simulink model "PMSM_PI_CONTROL"  (R2024b)
settings: Solver=ode4  StartTime=0.0  StopTime=2  FixedStep=Ts  RelTol=1e-3
InitFcn:
  | p=4;
  | RS=0.9585;
  | Rs=0.9585;
  | LS=0.00525;
  | Lq= 0.00525;
  | LAMDA_F=0.1827;
  | Ld=0.00525;
  | B=0.0003035;
  | J=0.0006329;
  | Vdc=300;
  | vcarp=150;
  | G=Vdc/(2*vcarp);
  | Ts = 1e-6;
  | kpi=2;
  | kii=100;
  | %% Current-loop bandwidth
  | f_ci = 100;        % Current controller bandwidth [Hz]
  | w_ci = 2*pi*f_ci;
  | 
  | %% d-axis PI
  | Kpd = Ld*w_ci;
  | Kid = Rs*w_ci;
  | 
  | %% q-axis PI
  | Kpq = Lq*w_ci;
  | Kiq = Rs*w_ci;
values from neighbouring files (symbols this model uses):
  phase = squeeze(phase)    [fir_filter.m]
  V = VPH - mean(VPH)    [three_level_inverter.m]
libraries: spsdq0toabcLib x2, spsabctoAlphaBetaZeroLib x2, spsabctodq0Lib x1, spsPermanentMagnetSynchronousMachineLib x1, spspowerguiLib x1, slpidlib x1
settings Model: SimulationMode=accelerator  Creator=killa  LastModifiedBy=killa

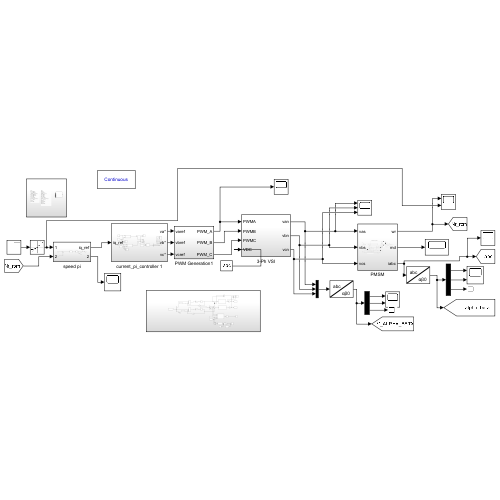
[thumbnail: Simulink's stored preview of the top-level diagram]
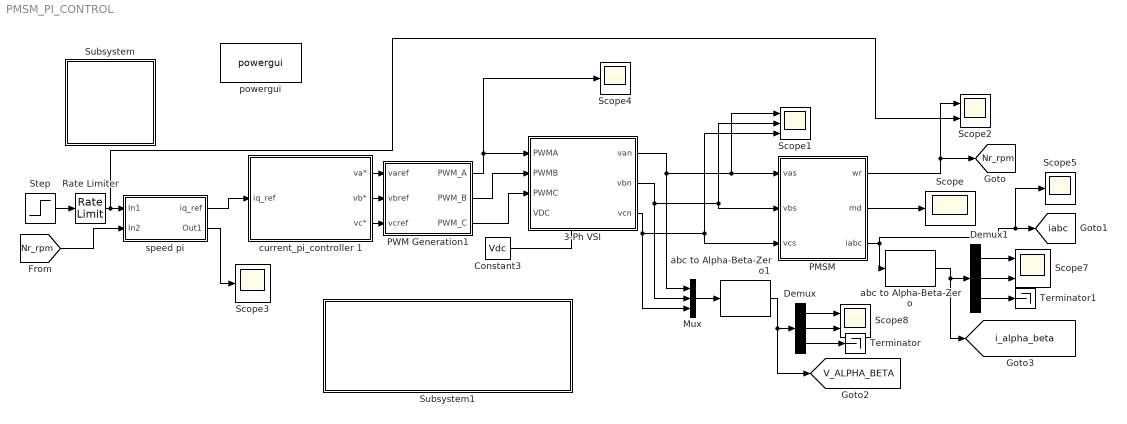
== system PMSM_PI_CONTROL ==
  3-Ph VSI : Subsystem
  Constant3 : Constant  Value=Vdc
  Demux : Demux  Outputs=3
  Demux1 : Demux  Outputs=3
  Mux : Mux  Inputs=3
  PMSM : Subsystem
  PWM Generation1 : Subsystem
  Rate Limiter : RateLimiter  RisingSlewLimit=10000  FallingSlewLimit=-10000
  Scope{,3..5} (4 alike) : Scope
  Scope1 : Scope  NumInputPorts=3
  Scope2 : Scope  NumInputPorts=2
  Scope7 : Scope  NumInputPorts=2
  Scope8 : Scope  NumInputPorts=2
  Step : Step  Before=500  After=1000  SampleTime=0
  Subsystem : Subsystem
  Subsystem1 : Subsystem
  Terminator : Terminator
  Terminator1 : Terminator
  abc to Alpha-Beta-Zero : spsabctoAlphaBetaZeroLib/abc to Alpha-Beta-Zero
  abc to Alpha-Beta-Zero1 : spsabctoAlphaBetaZeroLib/abc to Alpha-Beta-Zero
  current_pi_controller 1 : Subsystem
  powergui : spspowerguiLib/powergui  Priority=1  SimulationMode=Continuous  SampleTime=50e-6  frequency=60  Iterations=50  frequencyindice=60  Pbase=100e6  ErrMax=1e-4  UnitsV=kV  UnitsW=MW  buscounter=0  FunctionMessages=off  echomessages=off  EnableUseOfTLC=off  CurrentSourceSwitches=off  DisableSnubberDevices=off  DisableRonSwitches=off  DisableVfSwitches=off  DisplayEquations=off  AutomaticDiscreteSolvers=off  SolverType=Tustin/Backward Euler (TBE)  Interpol=off  ExternalGateDelay=off  methode=off  Ts=100  x0status=blocks  SPID=on  SwTol=0  HookPort=off  NonlinearTolerance=1e-4  nMaxIteration=100  ContinueOnMaxIteration=off  RestoreLinks=warning  ResistiveCurrentMeasurement=off  Frange=[0:2:500]  Ylog=off  Xlog=on  ShowGrid=off  save=off  variable=ZData  structure=0  ZoomFFT=off  StartTime=0.0  cycles=1  DisplayStyle=1  fundamental=60  FreqAxis=off  MaxFrequency=1000  frequencyindicesteady=1  RmsSteady=1  display=off
  speed pi : Subsystem
  tag scope: Nr_rpm=global, V_ALPHA_BETA=global, i_alpha_beta=global, iabc=global
  wires:
  PWM Generation1/1(PWM_A) -> Scope4/1, 3-Ph VSI/1(PWMA)
  speed pi/1(iq_ref) -> current_pi_controller 1/1(iq_ref)
  speed pi/2(Out1) -> Scope3/1
  Step/1 -> Rate Limiter/1
  Constant3/1 -> 3-Ph VSI/4(VDC)
  [Nr_rpm] -> speed pi/2(In2)
  PMSM/1(wr) -> [Nr_rpm], Scope2/1
  3-Ph VSI/3(vcn) -> Mux/3, PMSM/3(vcs), Scope1/3
  PWM Generation1/3(PWM_C) -> 3-Ph VSI/3(PWMC)
  PWM Generation1/2(PWM_B) -> 3-Ph VSI/2(PWMB)
  3-Ph VSI/1(van) -> PMSM/1(vas), Scope1/1, Mux/1
  current_pi_controller 1/1(va*) -> PWM Generation1/1(varef)
  current_pi_controller 1/3(vc*) -> PWM Generation1/3(vcref)
  current_pi_controller 1/2(vb*) -> PWM Generation1/2(vbref)
  PMSM/3(iabc) -> Scope5/1, [iabc], abc to Alpha-Beta-Zero/1
  PMSM/2(md) -> Scope/1
  Mux/1 -> abc to Alpha-Beta-Zero1/1
  3-Ph VSI/2(vbn) -> Mux/2, PMSM/2(vbs), Scope1/2
  Demux/1 -> Scope8/1
  Demux/2 -> Scope8/2
  abc to Alpha-Beta-Zero/1 -> [i_alpha_beta], Demux1/1
  Demux1/1 -> Scope7/1
  Demux1/2 -> Scope7/2
  Demux/3 -> Terminator/1
  Demux1/3 -> Terminator1/1
  abc to Alpha-Beta-Zero1/1 -> [V_ALPHA_BETA], Demux/1
  Rate Limiter/1 -> Scope2/2, speed pi/1(In1)

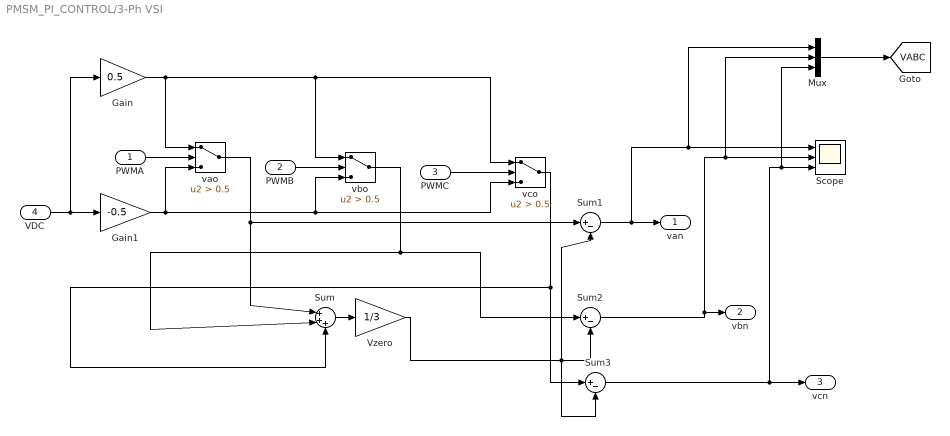
== system PMSM_PI_CONTROL/3-Ph VSI ==
  PWMA : Inport
  PWMB : Inport  Port=2
  PWMC : Inport  Port=3
  VDC : Inport  Port=4
  Gain : Gain  Gain=0.5
  Gain1 : Gain  Gain=-0.5
  Mux : Mux  Inputs=3
  Scope : Scope  NumInputPorts=3
  Sum : Sum  Inputs=|+++
  Sum1 : Sum  Inputs=|+-
  Sum2 : Sum  Inputs=|+-
  Sum3 : Sum  Inputs=|+-
  Vzero : Gain  Gain=1/3
  vao : Switch  Criteria=u2 > Threshold  Threshold=0.5  SaturateOnIntegerOverflow=off  InputSameDT=off
  vbo : Switch  Criteria=u2 > Threshold  Threshold=0.5  SaturateOnIntegerOverflow=off  InputSameDT=off
  vco : Switch  Criteria=u2 > Threshold  Threshold=0.5  SaturateOnIntegerOverflow=off  InputSameDT=off
  van : Outport
  vbn : Outport  Port=2
  vcn : Outport  Port=3
  tag scope: VABC=global
  wires:
  Gain/1 -> vao/1, vbo/1, vco/1
  Gain1/1 -> vao/3, vbo/3, vco/3
  VDC/1 -> Gain/1, Gain1/1
  PWMA/1 -> vao/2
  PWMB/1 -> vbo/2
  PWMC/1 -> vco/2
  vbo/1 -> Sum/2, Sum2/1
  vco/1 -> Sum/3, Sum3/1
  Sum/1 -> Vzero/1
  vao/1 -> Sum/1, Sum1/1
  Sum1/1 -> Mux/1, Scope/1, van/1
  Sum2/1 -> Mux/2, Scope/2, vbn/1
  Sum3/1 -> Mux/3, Scope/3, vcn/1
  Vzero/1 -> Sum3/2, Sum2/2, Sum1/2
  Mux/1 -> [VABC]

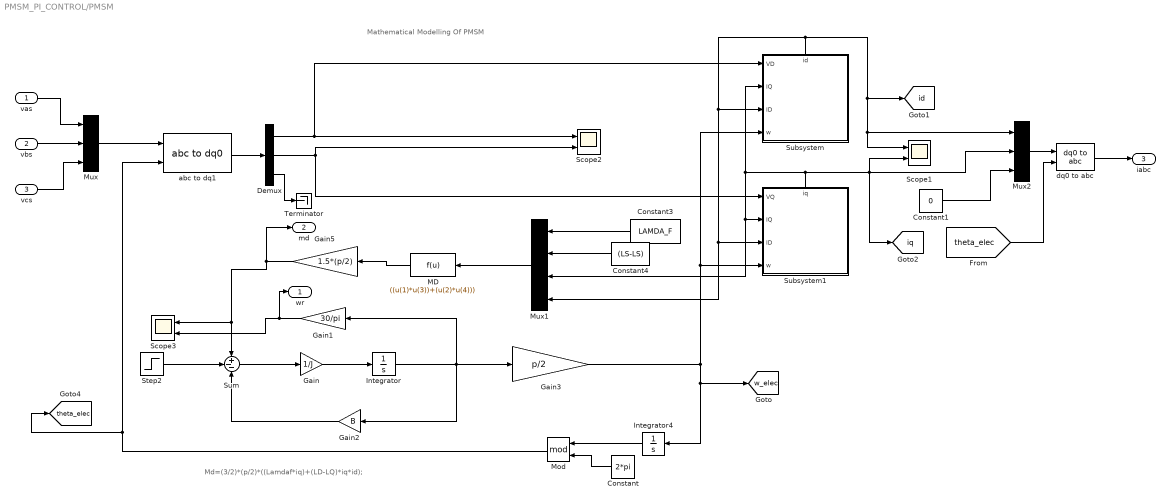
== system PMSM_PI_CONTROL/PMSM ==
  note: Mathematical Modelling Of PMSM
  note: Md=(3/2)*(p/2)*((Lamdaf*iq)+(LD-LQ)*iq*id);
  vas : Inport
  vbs : Inport  Port=2
  vcs : Inport  Port=3
  Constant : Constant  Value=2*pi
  Constant1 : Constant  Value=0
  Constant3 : Constant  Value=LAMDA_F
  Constant4 : Constant  Value=(LS-LS)
  Demux : Demux  Outputs=3
  Gain : Gain  Gain=1/J
  Gain1 : Gain  Gain=30/pi
  Gain2 : Gain  Gain=B
  Gain3 : Gain  Gain=p/2
  Gain5 : Gain  Gain=1.5*(p/2)
  Integrator : Integrator
  Integrator4 : Integrator
  MD : Fcn  Expr=((u(1)*u(3))+(u(2)*u(4)))
  Mod : Math  Operator=mod
  Mux : Mux  Inputs=3
  Mux1 : Mux
  Mux2 : Mux  Inputs=3
  Scope1 : Scope  NumInputPorts=2
  Scope2 : Scope  NumInputPorts=2
  Scope3 : Scope  NumInputPorts=2
  Step2 : Step  Time=0.5  Before=1  After=5  SampleTime=0
  Subsystem : Subsystem
      settings: PortSchema="{\"entries\":[{\"content\":{\"sides\":[{\"content\":{\"connectorIds\":[\"In1\",\"In2\",\"In3\",\"In4\"]},\"type\":\"ConnectorPlacement.EquallySpacedRectSide\",\"uuid\":\"8bdfacbe-4a3a-4ee8-bd8b-fd9f165566ad\"},{\"content\":{\"side\":\"RIGHT\"},\"type\":\"ConnectorPlacement.EquallySpacedRectSide\",\"uuid\":\"d7d447ea-68c0-4048-9ad9-b0a4b9da88db\"},{\"content\":{\"connectorIds\":[\"Out1\"],\"side\":\"TOP\"},\"type\":\"ConnectorPlacement.EquallySpacedRectSide\",\"uuid\":\"b7ac2ad5-65e5-4d40-8b7d-b38f0c69dbd3\"}]},\"type\":\"ConnectorPlacement.EquallySpacedConnector\",\"uuid\":\"b233c12a-b13d-4732-89f8-f9fe229221af\"}],\"packageUris\":[\"http://schema.mathworks.com/mf0/Connector/R2020b\"],\"version\":\"1.0\"}"
  Subsystem1 : Subsystem
      settings: PortSchema="{\"entries\":[{\"content\":{\"sides\":[{\"content\":{\"connectorIds\":[\"In1\",\"In2\",\"In3\",\"In4\"]},\"type\":\"ConnectorPlacement.EquallySpacedRectSide\",\"uuid\":\"6a02ce95-2547-4019-ba1c-0297980e75c1\"},{\"content\":{\"side\":\"RIGHT\"},\"type\":\"ConnectorPlacement.EquallySpacedRectSide\",\"uuid\":\"b1a391f9-ac05-4a60-810a-c34cda090cbe\"},{\"content\":{\"connectorIds\":[\"Out1\"],\"side\":\"TOP\"},\"type\":\"ConnectorPlacement.EquallySpacedRectSide\",\"uuid\":\"b02dfd25-1f32-4ddc-a79d-3ed5d594643e\"}]},\"type\":\"ConnectorPlacement.EquallySpacedConnector\",\"uuid\":\"98d8064c-9ae1-4c8d-8330-54a5e7664553\"}],\"packageUris\":[\"http://schema.mathworks.com/mf0/Connector/R2020b\"],\"version\":\"1.0\"}"
  Sum : Sum  Inputs=+--
  Terminator : Terminator
  abc to dq1 : spsabctodq0Lib/abc to dq0  Alignment=90 degrees behind phase A axis
  dq0 to abc : spsdq0toabcLib/dq0 to abc  Alignment=90 degrees behind phase A axis
  wr : Outport
  md : Outport  Port=2
  iabc : Outport  Port=3
  tag scope: id=global, iq=global, theta_elec=global, w_elec=global
  wires:
  Gain3/1 -> [w_elec], Integrator4/1, Subsystem/4(w), Subsystem1/4(w)
  Gain1/1 -> wr/1, Scope3/2
  Subsystem/1(id) -> [id], Mux2/1, Scope1/1, Mux1/4, Subsystem1/3(ID), Subsystem/3(ID)
  Gain2/1 -> Sum/3
  Demux/1 -> Scope2/1, Subsystem/1(VD)
  abc to dq1/1 -> Demux/1
  Step2/1 -> Sum/2
  Integrator/1 -> Gain2/1, Gain3/1, Gain1/1
  Subsystem1/1(iq) -> [iq], Mux2/2, Scope1/2, Subsystem/2(IQ), Mux1/3, Subsystem1/2(IQ)
  Integrator4/1 -> Mod/1
  Constant3/1 -> Mux1/1
  MD/1 -> Gain5/1
  Mux1/1 -> MD/1
  Constant/1 -> Mod/2
  Demux/3 -> Terminator/1
  Gain5/1 -> Scope3/1, Sum/1, md/1
  Gain/1 -> Integrator/1
  Sum/1 -> Gain/1
  Demux/2 -> Scope2/2, Subsystem1/1(VQ)
  Constant4/1 -> Mux1/2
  Mux/1 -> abc to dq1/1
  vas/1 -> Mux/1
  vbs/1 -> Mux/2
  vcs/1 -> Mux/3
  Mux2/1 -> dq0 to abc/1
  Constant1/1 -> Mux2/3
  [theta_elec] -> dq0 to abc/2
  dq0 to abc/1 -> iabc/1
  Mod/1 -> [theta_elec], abc to dq1/2

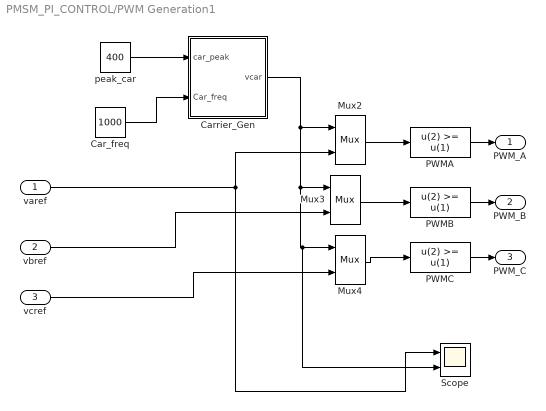
== system PMSM_PI_CONTROL/PWM Generation1 ==
  varef : Inport
  vbref : Inport  Port=2
  vcref : Inport  Port=3
  Car_freq : Constant  Value=1000
  Carrier_Gen : Subsystem
  Mux2 : Mux  Inputs=2
  Mux3 : Mux  Inputs=2
  Mux4 : Mux  Inputs=2
  PWMA : Fcn  Expr=u(2) >= u(1)
  PWMB : Fcn  Expr=u(2) >= u(1)
  PWMC : Fcn  Expr=u(2) >= u(1)
  Scope : Scope  NumInputPorts=2
  peak_car : Constant  Value=400
  PWM_A : Outport
  PWM_B : Outport  Port=2
  PWM_C : Outport  Port=3
  wires:
  varef/1 -> Mux2/2, Scope/1
  Car_freq/1 -> Carrier_Gen/2(Car_freq)
  peak_car/1 -> Carrier_Gen/1(car_peak)
  vcref/1 -> Mux4/2
  PWMC/1 -> PWM_C/1
  vbref/1 -> Mux3/2
  PWMB/1 -> PWM_B/1
  PWMA/1 -> PWM_A/1
  Mux4/1 -> PWMC/1
  Mux3/1 -> PWMB/1
  Mux2/1 -> PWMA/1
  Carrier_Gen/1(vcar) -> Mux2/1, Mux3/1, Mux4/1, Scope/2

== system PMSM_PI_CONTROL/Subsystem ==
  note: p=4;
      | RS=0.9585;
      | LS=0.00525;
      | LAMDA_F=0.1827;
      | B=0.0003035;
      | J=0.0006329;
      | Vdc=300;
      | vcarp=150;
      | G=Vdc/(2*vcarp);
      | Ts = 1e-6;
      | kpi=2;
      | kii=100;
  note: p=8;
      | RS=30;
      | LS=50e-3;
      | LAMDA_F=0.2;
      | B=0.0003;
      | J=0.002;
      | Vdc=400;
      | vcarp=150;
      | G=Vdc/(2*vcarp);
      | Ts = 1e-6;
      | kpid=2;
      | kiid=100;
      | kpiq=2;
      | kiiq=100;
  Permanent Magnet Synchronous Machine : spsPermanentMagnetSynchronousMachineLib/Permanent Magnet Synchronous Machine  Commented=on  NbPhases=3  FluxDistribution=Sinusoidal  RotorType=Round  MechanicalLoad=Torque Tm  PresetModel="05:  8 Nm 300 Vdc 2000 RPM - 10 Nm"  ShowDetailedParameters=on  MeasurementBus=off  Resistance=0.9585  Inductance=8.5e-3  dqInductances=[8.5e-3,8.5e-3]  La=0.00525  MachineConstant=Flux linkage established by magnets (V.s)  Flux=0.1827  VoltageCst=132.5525  TorqueCst=1.0962  Flat=120  Mechanical=[0.0006329 0.0003035 4 0]  PolePairs=4  InitialConditions=[0,0, 0,0]  InitialConditions5ph=[0 0 0 0 0 0]  RefAngle=90 degrees behind phase A axis (modified Park)  IterativeDiscreteModel=Trapezoidal non iterative  TsBlock=-1  TsPowergui=0

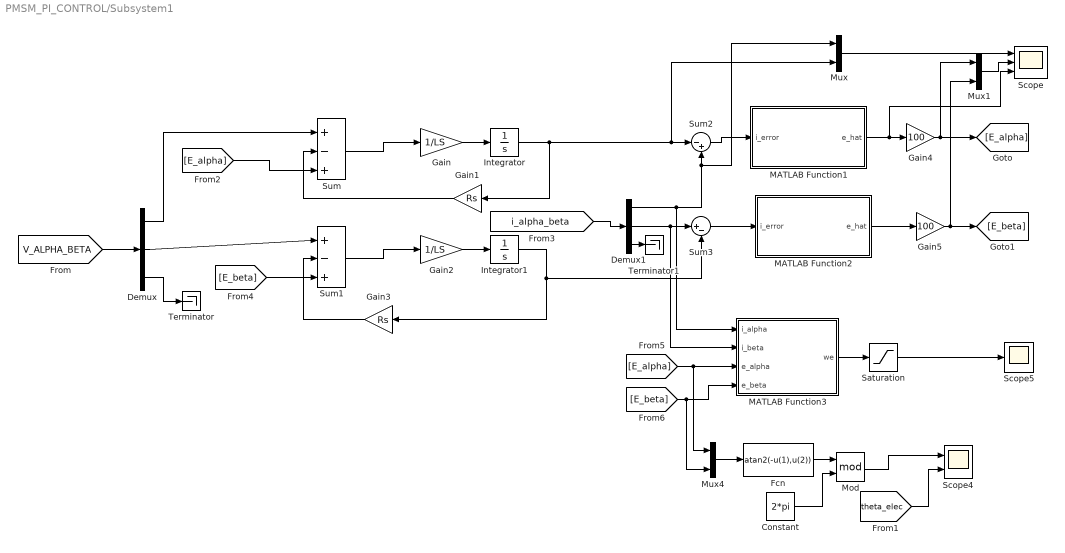
== system PMSM_PI_CONTROL/Subsystem1 ==
  Constant : Constant  Value=2*pi
  Demux : Demux  Outputs=3
  Demux1 : Demux  Outputs=3
  Fcn : Fcn  Expr=atan2(-u(1),u(2))
  Gain : Gain  Gain=1/LS
  Gain1 : Gain  Gain=Rs
  Gain2 : Gain  Gain=1/LS
  Gain3 : Gain  Gain=Rs
  Gain4 : Gain  Gain=100
  Gain5 : Gain  Gain=100
  Integrator : Integrator
  Integrator1 : Integrator
  MATLAB Function1 : MATLAB Function  TreatAsAtomicUnit=on
  MATLAB Function2 : MATLAB Function  TreatAsAtomicUnit=on
  MATLAB Function3 : MATLAB Function  TreatAsAtomicUnit=on
  Mod : Math  Operator=mod
  Mux : Mux  Inputs=2
  Mux1 : Mux  Inputs=2
  Mux4 : Mux  Inputs=2
  Saturation : Saturate  UpperLimit=5000  LowerLimit=-5000
  Scope : Scope  NumInputPorts=3
  Scope4 : Scope  NumInputPorts=2
  Scope5 : Scope
  Sum : Sum  Inputs=|+-+
  Sum1 : Sum  Inputs=|+-+
  Sum2 : Sum  Inputs=|-+
  Sum3 : Sum  Inputs=|+-
  Terminator : Terminator
  Terminator1 : Terminator
  wires:
  Fcn/1 -> Mod/1
  Constant/1 -> Mod/2
  MATLAB Function3/1(we) -> Saturation/1
  Mod/1 -> Scope4/1
  Mux4/1 -> Fcn/1
  [V_ALPHA_BETA] -> Demux/1
  Demux/3 -> Terminator/1
  Demux1/3 -> Terminator1/1
  [i_alpha_beta] -> Demux1/1
  Saturation/1 -> Scope5/1
  [theta_elec] -> Scope4/2
  Demux/1 -> Sum/1
  Sum/1 -> Gain/1
  Gain/1 -> Integrator/1
  Gain1/1 -> Sum/2
  Demux/2 -> Sum1/1
  Integrator1/1 -> Sum3/2, Gain3/1
  Gain2/1 -> Integrator1/1
  Sum1/1 -> Gain2/1
  Gain3/1 -> Sum1/2
  Demux1/1 -> MATLAB Function3/1(i_alpha), Mux/1, Sum2/2
  Demux1/2 -> MATLAB Function3/2(i_beta), Sum3/1
  Sum2/1 -> MATLAB Function1/1(i_error)
  Sum3/1 -> MATLAB Function2/1(i_error)
  MATLAB Function1/1(e_hat) -> Scope/3, Gain4/1
  MATLAB Function2/1(e_hat) -> Gain5/1
  Gain4/1 -> Mux1/1, [E_alpha]
  Gain5/1 -> [E_beta], Mux1/2
  [E_alpha] -> MATLAB Function3/3(e_alpha), Mux4/1
  [E_beta] -> Mux4/2, MATLAB Function3/4(e_beta)
  Mux/1 -> Scope/1
  Integrator/1 -> Mux/2, Sum2/1, Gain1/1
  Mux1/1 -> Scope/2
  [E_alpha] -> Sum/3
  [E_beta] -> Sum1/3

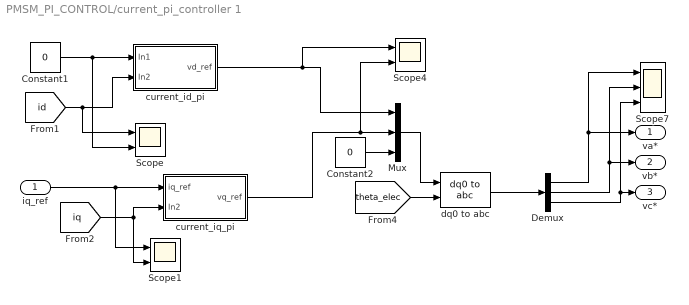
== system PMSM_PI_CONTROL/current_pi_controller 1 ==
  iq_ref : Inport
  Constant1 : Constant  Value=0
  Constant2 : Constant  Value=0
  Demux : Demux  Outputs=3
  Mux : Mux  Inputs=3
  Scope : Scope  NumInputPorts=2
  Scope1 : Scope  NumInputPorts=2
  Scope4 : Scope  NumInputPorts=2
  Scope7 : Scope  NumInputPorts=3
  current_id_pi : Subsystem
  current_iq_pi : Subsystem
  dq0 to abc : spsdq0toabcLib/dq0 to abc  Alignment=90 degrees behind phase A axis
  va* : Outport
  vb* : Outport  Port=2
  vc* : Outport  Port=3
  wires:
  Demux/3 -> vc*/1, Scope7/3
  Demux/2 -> vb*/1, Scope7/2
  Demux/1 -> va*/1, Scope7/1
  dq0 to abc/1 -> Demux/1
  [theta_elec] -> dq0 to abc/2
  iq_ref/1 -> Scope1/1, current_iq_pi/1(iq_ref)
  [iq] -> current_iq_pi/2(In2), Scope1/2
  Constant2/1 -> Mux/3
  [id] -> current_id_pi/2(In2), Scope/1
  Mux/1 -> dq0 to abc/1
  Constant1/1 -> Scope/2, current_id_pi/1(In1)
  current_id_pi/1(vd_ref) -> Scope4/1, Mux/1
  current_iq_pi/1(vq_ref) -> Scope4/2, Mux/2

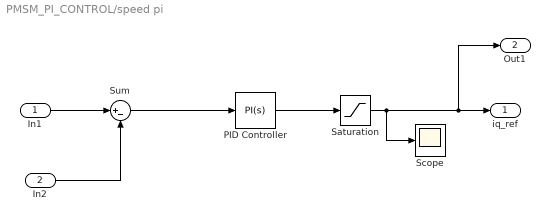
== system PMSM_PI_CONTROL/speed pi ==
  In1 : Inport
  In2 : Inport  Port=2
  PID Controller : slpidlib/PID Controller  Controller=PI  Form=Parallel  TimeDomain=Continuous-time  UseExternalTs=off  SampleTime=-1  IntegratorMethod=Forward Euler  FilterMethod=Forward Euler  ControllerParametersSource=internal  P=0.1  I=2  UseKiTs=off  D=0  UseExternalDerivativeSource=off  N=100  UseFilter=on  TunerSelectOption=Transfer Function Based (PID Tuner App)  InitialConditionSource=internal  InitialConditionForIntegrator=0  InitialConditionForFilter=0  DifferentiatorICPrevScaledInput=0  ExternalReset=none  TrackingMode=off  Kt=1  LimitOutput=off  SatLimitsSource=internal  UpperSaturationLimit=80  LowerSaturationLimit=-40  LinearizeAsGain=on  AntiWindupMode=clamping  Kb=1  LimitIntegrator=off  UpperIntegratorSaturationLimit=inf  LowerIntegratorSaturationLimit=-inf  POutMin=[]  POutMax=[]  IOutMin=[]  IOutMax=[]  DOutMin=[]  DOutMax=[]  NOutMin=[]  NOutMax=[]  SumOutMin=[]  SumOutMax=[]  SaturationOutMin=[]  SaturationOutMax=[]  PParamMin=[]  PParamMax=[]  IParamMin=[]  IParamMax=[]  DParamMin=[]  DParamMax=[]  NParamMin=[]  NParamMax=[]  KbParamMin=[]  KbParamMax=[]  KtParamMin=[]  KtParamMax=[]  KbOutMin=[]  KbOutMax=[]  KtOutMin=[]  KtOutMax=[]  IntegratorOutMin=[]  IntegratorOutMax=[]  FilterOutMin=[]  FilterOutMax=[]  SumI1OutMin=[]  SumI1OutMax=[]  SumI2OutMin=[]  SumI2OutMax=[]  SumI3OutMin=[]  SumI3OutMax=[]  SumI4OutMin=[]  SumI4OutMax=[]  SumDOutMin=[]  SumDOutMax=[]  DifferentiatorOutMin=[]  DifferentiatorOutMax=[]  FilterDiffOutCoefMin=[]  FilterDiffOutCoefMax=[]  ReciprocalOutMin=[]  ReciprocalOutMax=[]  SumDenOutMin=[]  SumDenOutMax=[]  SumNumOutMin=[]  SumNumOutMax=[]  DivideOutMin=[]  DivideOutMax=[]  UdiffTsProdOutMin=[]  UdiffTsProdOutMax=[]  NTsProdOutMin=[]  NTsProdOutMax=[]  UintegralTsProdOutMin=[]  UintegralTsProdOutMax=[]  UngainTsProdOutMin=[]  UngainTsProdOutMax=[]  ClampingZeroOutDataTypeStr=Inherit: Inherit via back propagation  ClampingZeroOutMin=[]  ClampingZeroOutMax=[]  FilterDenConstantOutDataTypeStr=Inherit: Inherit via back propagation  FilterDenConstantOutMin=[]  FilterDenConstantOutMax=[]  PCopyOutDataTypeStr=Inherit: Inherit via back propagation  PCopyOutMin=[]  PCopyOutMax=[]  NCopyOutDataTypeStr=Inherit: Inherit via back propagation  NCopyOutMin=[]  NCopyOutMax=[]  IntegratorContinuousStateAttributes=''  IntegratorStateMustResolveToSignalObject=off  IntegratorRTWStateStorageClass=Auto  FilterContinuousStateAttributes=''  FilterStateMustResolveToSignalObject=off  FilterRTWStateStorageClass=Auto  ParallelPVariant=InternalParameters  IdealPVariant=Disabled  IVariant=InternalParameters  DVariant=Disabled  IntegratorVariant=Continuous  SatVariant=Disabled  AWVariant=Passthrough  PCopyVariant=Disabled  TRVariant=Disabled  FdbkBlocksVariant=Forward  IdealPFdbkVariant=Disabled  SatFdbkVariant=Disabled  DerivativeFilterVariant=Disabled  NVariant=Disabled  NCopyVariant=Disabled_SignalSpec  FilterICVariant=Disabled  IntegratorICVariant=InternalICs  ExternalResetVariant=Disabled  TRSumVariant=Passthrough  SumFdbkVariant=Disabled  SumVariant=Sum_PI  TsampFilterVariant=InternalTs  TsampNgainVariant=Passthrough  TsampIntegralVariant=Disabled_SignalSpec  ExternalSaturationOutDataTypeStr=Inherit: Same as second input  DerivativeSourceVariant=Disabled  PreIntVariant=InternalPreInt
  Saturation : Saturate  UpperLimit=12  LowerLimit=-12
  Scope : Scope
  Sum : Sum  Inputs=|+-
  iq_ref : Outport
  Out1 : Outport  Port=2
  wires:
  In1/1 -> Sum/1
  In2/1 -> Sum/2
  PID Controller/1 -> Saturation/1
  Sum/1 -> PID Controller/1
  Saturation/1 -> Scope/1, Out1/1, iq_ref/1

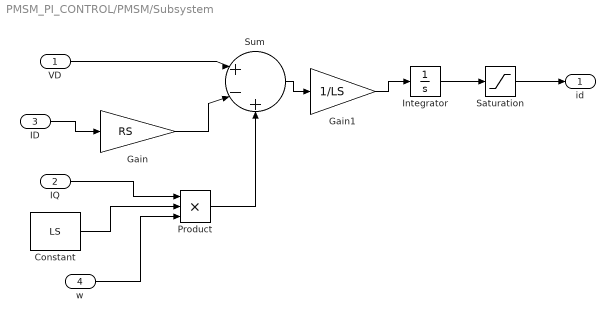
== system PMSM_PI_CONTROL/PMSM/Subsystem ==
  VD : Inport
  IQ : Inport  Port=2
  ID : Inport  Port=3
  w : Inport  Port=4
  Constant : Constant  Value=LS
  Gain : Gain  Gain=RS
  Gain1 : Gain  Gain=1/LS
  Integrator : Integrator
  Product : Product  Inputs=3
  Saturation : Saturate  UpperLimit=40  LowerLimit=-40
  Sum : Sum  Inputs=|+-+
  id : Outport
  wires:
  VD/1 -> Sum/1
  ID/1 -> Gain/1
  Gain/1 -> Sum/2
  IQ/1 -> Product/1
  w/1 -> Product/3
  Constant/1 -> Product/2
  Product/1 -> Sum/3
  Sum/1 -> Gain1/1
  Integrator/1 -> Saturation/1
  Gain1/1 -> Integrator/1
  Saturation/1 -> id/1

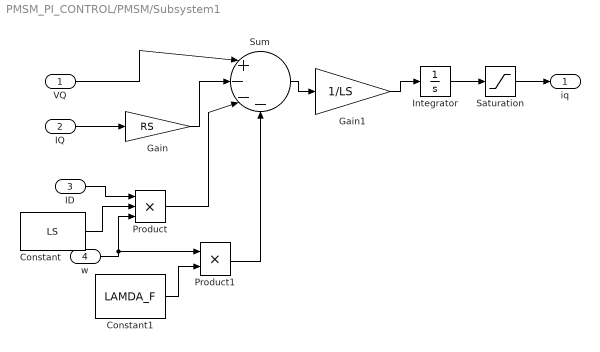
== system PMSM_PI_CONTROL/PMSM/Subsystem1 ==
  VQ : Inport
  IQ : Inport  Port=2
  ID : Inport  Port=3
  w : Inport  Port=4
  Constant : Constant  Value=LS
  Constant1 : Constant  Value=LAMDA_F
  Gain : Gain  Gain=RS
  Gain1 : Gain  Gain=1/LS
  Integrator : Integrator  UpperSaturationLimit=100  LowerSaturationLimit=-100
  Product : Product  Inputs=3
  Product1 : Product
  Saturation : Saturate  UpperLimit=50  LowerLimit=-50
  Sum : Sum  Inputs=|+---
  iq : Outport
  wires:
  Integrator/1 -> Saturation/1
  Sum/1 -> Gain1/1
  Product/1 -> Sum/3
  Constant/1 -> Product/2
  Gain/1 -> Sum/2
  VQ/1 -> Sum/1
  IQ/1 -> Gain/1
  Gain1/1 -> Integrator/1
  ID/1 -> Product/1
  w/1 -> Product1/1, Product/3
  Constant1/1 -> Product1/2
  Product1/1 -> Sum/4
  Saturation/1 -> iq/1

== system PMSM_PI_CONTROL/PWM Generation1/Carrier_Gen ==
  car_peak : Inport
  Car_freq : Inport  Port=2
  Scope1 : Scope
  carrier : Subsystem
  vcar : Outport
  wires:
  Car_freq/1 -> carrier/1(In1)
  carrier/1(Out1) -> vcar/1, Scope1/1
  car_peak/1 -> carrier/2(In2)

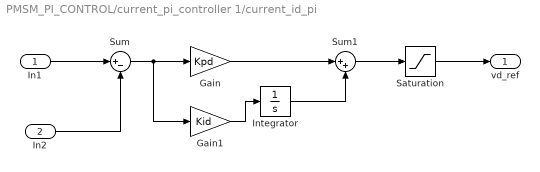
== system PMSM_PI_CONTROL/current_pi_controller 1/current_id_pi ==
  In1 : Inport
  In2 : Inport  Port=2
  Gain : Gain  Gain=Kpd
  Gain1 : Gain  Gain=Kid
  Integrator : Integrator  LimitOutput=on
  Saturation : Saturate  UpperLimit=200  LowerLimit=-200
  Sum : Sum  Inputs=|+-
  Sum1 : Sum  Inputs=|++
  vd_ref : Outport
  wires:
  Sum1/1 -> Saturation/1
  Sum/1 -> Gain1/1, Gain/1
  Gain/1 -> Sum1/1
  Integrator/1 -> Sum1/2
  Gain1/1 -> Integrator/1
  In1/1 -> Sum/1
  In2/1 -> Sum/2
  Saturation/1 -> vd_ref/1

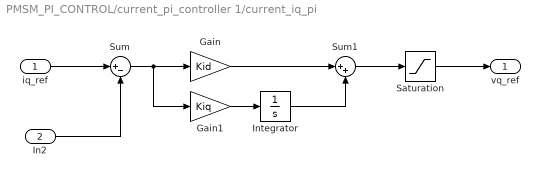
== system PMSM_PI_CONTROL/current_pi_controller 1/current_iq_pi ==
  iq_ref : Inport
  In2 : Inport  Port=2
  Gain : Gain  Gain=Kid
  Gain1 : Gain  Gain=Kiq
  Integrator : Integrator  LimitOutput=on
  Saturation : Saturate  UpperLimit=200  LowerLimit=-200
  Sum : Sum  Inputs=|+-
  Sum1 : Sum  Inputs=|++
  vq_ref : Outport
  wires:
  Saturation/1 -> vq_ref/1
  In2/1 -> Sum/2
  iq_ref/1 -> Sum/1
  Gain1/1 -> Integrator/1
  Integrator/1 -> Sum1/2
  Gain/1 -> Sum1/1
  Sum/1 -> Gain/1, Gain1/1
  Sum1/1 -> Saturation/1

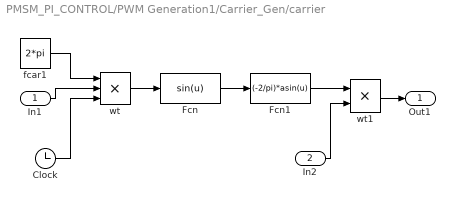
== system PMSM_PI_CONTROL/PWM Generation1/Carrier_Gen/carrier ==
  In1 : Inport
  In2 : Inport  Port=2
  Clock : Clock
  Fcn : Fcn  Expr=sin(u)
  Fcn1 : Fcn  Expr=(-2/pi)*asin(u)
  fcar1 : Constant  Value=2*pi
  wt : Product  Inputs=3  RndMeth=Zero
  wt1 : Product  RndMeth=Zero
  Out1 : Outport
  wires:
  In2/1 -> wt1/2
  wt1/1 -> Out1/1
  In1/1 -> wt/2
  Fcn1/1 -> wt1/1
  Fcn/1 -> Fcn1/1
  wt/1 -> Fcn/1
  Clock/1 -> wt/3
  fcar1/1 -> wt/1

== matlab function PMSM_PI_CONTROL/Subsystem1/MATLAB Function2 ==
  data: i_error input; e_hat output
function e_hat = fcn(i_error)


% Observer Parameters      % Observer gain
a  = 1;    % Smoothing parameter
n  = 1;        % Nonlinearity exponent

% Soft-Sign Function
e_hat = ( i_error / (a + abs(i_error)^n) );

end

== matlab function PMSM_PI_CONTROL/Subsystem1/MATLAB Function1 ==
  data: i_error input; e_hat output
function e_hat = fcn(i_error)


%Observer Parameters      % Observer gain
a  = 1;    % Smoothing parameter
n  = 1;        % Nonlinearity exponent

% Soft-Sign Function
e_hat = ( i_error / (a + abs(i_error)^n) );

end

== matlab function PMSM_PI_CONTROL/Subsystem1/MATLAB Function3 ==
  data: i_alpha input; i_beta input; e_alpha input; we output; e_beta input
function we = fcn(i_alpha,i_beta,e_alpha,e_beta)
%#codegen
%
% Inputs:
% e_alpha : Estimated alpha-axis back EMF
% e_beta  : Estimated beta-axis back EMF
% i_alpha : Alpha-axis current
% i_beta  : Beta-axis current
% psi     : Permanent magnet flux linkage (Wb)
%
% Output:
% we      : Electrical speed (rad/s)
psi = 0.1857;
% Avoid division by zero
eps = 1e-8;

% Numerator
num = (e_beta*i_alpha - e_alpha*i_beta);

% Denominator
den = psi*sqrt(i_alpha^2 + i_beta^2);

if den < eps
    we = 0;
else
    we = num/den;
end

end
